simulink model "Simulacioncorrec"  (R2019a)
settings: Solver=VariableStepAuto  StartTime=0.0  StopTime=10.0  RelTol=1e-3
undefined symbols (not defined in the file): A, B, C, den, E, F, K, kd1, kd2, kd3, Ke, ki, kp, num, q0, q1, q2, tm
libraries: simulink x1
settings Model: Creator=julia  LastModifiedBy=julia

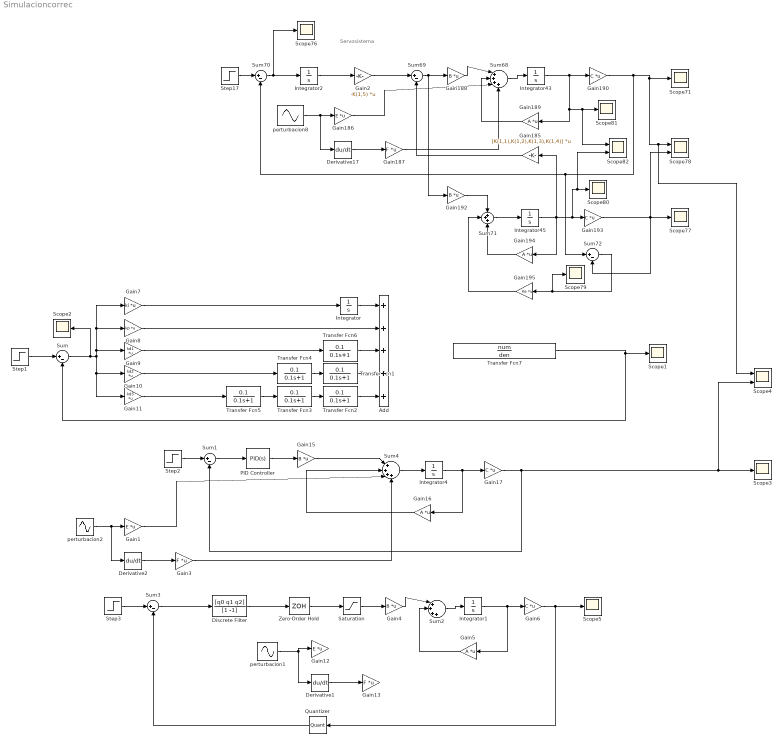
== system Simulacioncorrec ==
  note: Servosistema
  Add : Sum  Inputs=+++++
  Derivative1 : Derivative
  Derivative17 : Derivative
  Derivative2 : Derivative
  Discrete Filter : DiscreteFilter  Numerator=[q0 q1 q2]  Denominator=[1 -1]
  Gain1 : Gain  Gain=E  Multiplication=Matrix(K*u)
  Gain10 : Gain  Gain=kd2  Multiplication=Matrix(K*u)
  Gain11 : Gain  Gain=kd3  Multiplication=Matrix(K*u)
  Gain12 : Gain  Gain=E  Multiplication=Matrix(K*u)
  Gain13 : Gain  Gain=F  Multiplication=Matrix(K*u)
  Gain{4,15,188,192} (4 alike) : Gain  Gain=B  Multiplication=Matrix(K*u)
  Gain{5,16,189,194} (4 alike) : Gain  Gain=A  Multiplication=Matrix(K*u)
  Gain{6,17,190,193} (4 alike) : Gain  Gain=C  Multiplication=Matrix(K*u)
  Gain185 : Gain  Gain=[K(1,1),K(1,2),K(1,3),K(1,4)]  Multiplication=Matrix(K*u)
  Gain186 : Gain  Gain=E  Multiplication=Matrix(K*u)
  Gain187 : Gain  Gain=F  Multiplication=Matrix(K*u)
  Gain195 : Gain  Gain=Ke  Multiplication=Matrix(K*u)
  Gain2 : Gain  Gain=-K(1,5)  Multiplication=Matrix(K*u)
  Gain3 : Gain  Gain=F  Multiplication=Matrix(K*u)
  Gain7 : Gain  Gain=ki  Multiplication=Matrix(K*u)
  Gain8 : Gain  Gain=kp  Multiplication=Matrix(K*u)
  Gain9 : Gain  Gain=kd1  Multiplication=Matrix(K*u)
  Integrator{,1..2,4,43,45} (6 alike) : Integrator
  PID Controller : simulink/Continuous/PID Controller  Controller=PID  Form=Parallel  TimeDomain=Continuous-time  SampleTime=-1  IntegratorMethod=Forward Euler  FilterMethod=Forward Euler  ControllerParametersSource=internal  P=338.749200255715  I=64.9253571684444  D=383.35455629752  UseFilter=on  N=2.79652585685593  TunerSelectOption=Transfer Function Based (PID Tuner App)  InitialConditionSource=internal  InitialConditionForIntegrator=0  InitialConditionForFilter=0  DifferentiatorICPrevScaledInput=0  ExternalReset=none  TrackingMode=off  Kt=1  LimitOutput=off  UpperSaturationLimit=inf  LowerSaturationLimit=-inf  LinearizeAsGain=on  AntiWindupMode=none  Kb=1  POutMin=[]  POutMax=[]  IOutMin=[]  IOutMax=[]  DOutMin=[]  DOutMax=[]  NOutMin=[]  NOutMax=[]  SumOutMin=[]  SumOutMax=[]  SaturationOutMin=[]  SaturationOutMax=[]  PParamMin=[]  PParamMax=[]  IParamMin=[]  IParamMax=[]  DParamMin=[]  DParamMax=[]  NParamMin=[]  NParamMax=[]  KbParamMin=[]  KbParamMax=[]  KtParamMin=[]  KtParamMax=[]  KbOutMin=[]  KbOutMax=[]  KtOutMin=[]  KtOutMax=[]  IntegratorOutMin=[]  IntegratorOutMax=[]  FilterOutMin=[]  FilterOutMax=[]  SumI1OutMin=[]  SumI1OutMax=[]  SumI2OutMin=[]  SumI2OutMax=[]  SumI3OutMin=[]  SumI3OutMax=[]  SumI4OutMin=[]  SumI4OutMax=[]  SumDOutMin=[]  SumDOutMax=[]  DifferentiatorOutMin=[]  DifferentiatorOutMax=[]  FilterDiffOutCoefMin=[]  FilterDiffOutCoefMax=[]  ReciprocalOutMin=[]  ReciprocalOutMax=[]  SumDenOutMin=[]  SumDenOutMax=[]  SumNumOutMin=[]  SumNumOutMax=[]  DivideOutMin=[]  DivideOutMax=[]  IntegratorContinuousStateAttributes=''  IntegratorStateMustResolveToSignalObject=off  IntegratorRTWStateStorageClass=Auto  FilterContinuousStateAttributes=''  FilterStateMustResolveToSignalObject=off  FilterRTWStateStorageClass=Auto  ParallelPVariant=InternalParameters  IdealPVariant=Disabled  IVariant=InternalParameters  DVariant=InternalParameters  IntegratorVariant=Continuous  SatVariant=Disabled  AWVariant=Passthrough  PCopyVariant=Disabled  TRVariant=Disabled  FdbkBlocksVariant=Forward  IdealPFdbkVariant=Disabled  SatFdbkVariant=Disabled  DerivativeFilterVariant=ContFilter  NVariant=InternalParameters  NCopyVariant=Disabled  FilterICVariant=InternalICsFilter  IntegratorICVariant=InternalICs  ExternalResetVariant=Disabled  TRSumVariant=Passthrough  SumFdbkVariant=Disabled  SumVariant=Sum_PID
  Quantizer : Quantizer
  Saturation : Saturate
  Scope{1..3,5,71,76..77,79..81} (10 alike) : Scope
  Scope4 : Scope  NumInputPorts=2
  Scope78 : Scope  NumInputPorts=2
  Scope82 : Scope  NumInputPorts=2
  Step{1..3,17} (4 alike) : Step  Time=0  SampleTime=0
  Sum{,1,3,69..70,72} (6 alike) : Sum  Inputs=|+-
  Sum2 : Sum  Inputs=|++++
  Sum4 : Sum  Inputs=|++++
  Sum68 : Sum  Inputs=|++++
  Sum71 : Sum  Inputs=+++
  Transfer Fcn{1..6} (6 alike) : TransferFcn  Numerator=[0.1]  Denominator=[0.1 1]
  Transfer Fcn7 : TransferFcn  Numerator=num  Denominator=den
  Zero-Order Hold : ZeroOrderHold  SampleTime=tm
  perturbacion1 : Sin  Frequency=pi  SampleTime=0
  perturbacion2 : Sin  Frequency=pi  SampleTime=0
  perturbacion8 : Sin  Frequency=pi  SampleTime=0
  wires:
  Gain188/1 -> Sum68/1
  Derivative17/1 -> Gain187/1
  Step17/1 -> Sum70/1
  Gain185/1 -> Sum69/2
  Sum72/1 -> Scope79/1, Gain195/1
  Gain193/1 -> Sum72/2, Scope78/2, Scope77/1
  Gain195/1 -> Sum71/2
  Gain194/1 -> Sum71/3
  Integrator43/1 -> Scope82/1, Scope81/1, Gain189/1, Gain190/1
  Integrator45/1 -> Gain194/1, Gain185/1, Scope82/2, Scope80/1, Gain193/1
  Sum69/1 -> Gain192/1, Gain188/1
  Gain190/1 -> Sum72/1, Sum70/2, Scope4/1, Scope78/1, Scope71/1
  Gain192/1 -> Sum71/1
  Sum68/1 -> Integrator43/1
  Gain189/1 -> Sum68/2
  perturbacion8/1 -> Derivative17/1, Gain186/1
  Sum71/1 -> Integrator45/1
  Gain2/1 -> Sum69/1
  Integrator2/1 -> Gain2/1
  Sum70/1 -> Integrator2/1, Scope76/1
  Gain186/1 -> Sum68/3
  Gain187/1 -> Sum68/4
  Integrator/1 -> Add/1
  Gain8/1 -> Add/2
  Gain7/1 -> Integrator/1
  Transfer Fcn7/1 -> Sum/2, Scope1/1
  Sum/1 -> Scope2/1, Gain9/1, Gain7/1, Gain8/1, Gain11/1, Gain10/1
  Step1/1 -> Sum/1
  Transfer Fcn3/1 -> Transfer Fcn2/1
  Transfer Fcn5/1 -> Transfer Fcn3/1
  Transfer Fcn4/1 -> Transfer Fcn1/1
  Gain9/1 -> Transfer Fcn6/1
  Transfer Fcn6/1 -> Add/3
  Transfer Fcn1/1 -> Add/4
  Gain10/1 -> Transfer Fcn4/1
  Gain11/1 -> Transfer Fcn5/1
  Transfer Fcn2/1 -> Add/5
  PID Controller/1 -> Gain15/1
  Sum1/1 -> PID Controller/1
  Gain17/1 -> Sum1/2, Scope4/2, Scope3/1
  Step2/1 -> Sum1/1
  Gain15/1 -> Sum4/1
  Integrator4/1 -> Gain16/1, Gain17/1
  Sum4/1 -> Integrator4/1
  Gain16/1 -> Sum4/2
  Derivative2/1 -> Gain3/1
  perturbacion2/1 -> Derivative2/1, Gain1/1
  Gain3/1 -> Sum4/4
  Gain1/1 -> Sum4/3
  Gain5/1 -> Sum2/2
  Sum2/1 -> Integrator1/1
  Integrator1/1 -> Gain6/1, Gain5/1
  Gain4/1 -> Sum2/1
  perturbacion1/1 -> Gain12/1, Derivative1/1
  Derivative1/1 -> Gain13/1
  Gain6/1 -> Scope5/1, Quantizer/1
  Saturation/1 -> Gain4/1
  Zero-Order Hold/1 -> Saturation/1
  Quantizer/1 -> Sum3/2
  Sum3/1 -> Discrete Filter/1
  Step3/1 -> Sum3/1
  Discrete Filter/1 -> Zero-Order Hold/1
